simulink library "common_lib"  (R2015a)
settings: Solver=ode45  StartTime=0.0  StopTime=10.0  RelTol=1e-3
settings Model: Creator=SktUser15  LastModifiedBy=daysys

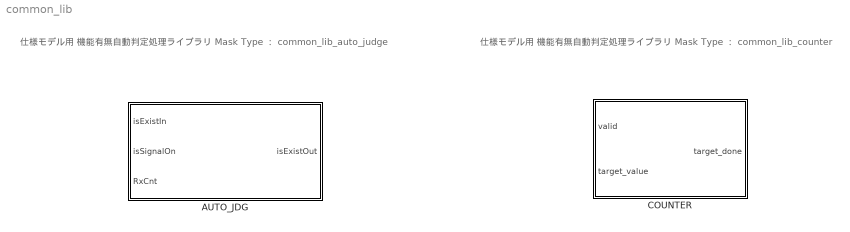
== system common_lib ==
  note: 仕様モデル用 機能有無自動判定処理ライブラリ
      | Mask Type ： common_lib_auto_judge
  note: 仕様モデル用 機能有無自動判定処理ライブラリ
      | Mask Type ： common_lib_counter
  AUTO_JDG : Subsystem  RequirementInfo={'other' '..\doc\SRS_Lib_AUTO_JDG.docx' '@Simulink_requirement_item_1' 'true' '[SRS_Lib_AUTO_JDG_Module _01-001]' '' ; 'other' '..\doc\SRS_Lib_AUTO_JDG.docx' '@Simulink_requirement_item_2' 'true' '[SRS_Lib_AUTO_JDG_Module _01-002]' '' ; 'other' '..\doc\SRS_Lib_AUTO_JDG.docx' '@Simulink_requirement_item_3' 'true' '[SRS_Lib_AUTO_JDG_Module _01-003]' '' ; 'other' '..\doc\SRS_Lib_AUTO_JDG.docx' '@Simulink_requirement_item_4' 'true' '[SRS_Lib_AUTO_JDG_Module _01-004]' '' ; 'other' '..\doc\SRS_Lib_AUTO_JDG.docx' '@Simulink_requirement_item_5' 'true' '[SRS_Lib_AUTO_JDG_Module _01-005]' '' ; 'other' '..\doc\SRS_Lib_AUTO_JDG.docx' '@Simulink_requirement_item_6' 'true' '[SRS_Lib_AUTO_JDG_Module _01-006]' '' ; 'other' '..\doc\SRS_Lib_AUTO_JDG.docx' '@Simulink_requirement_item_7' 'true' '[SRS_Lib_AUTO_JDG_Module _01-007]' '' ; 'other' '..\doc\SRS_Lib_AUTO_JDG.docx' '@Simulink_requirement_item_8' 'true' '[SRS_Lib_AUTO_JDG_Module _01-008]' '' ; 'other' '..\doc\SRS_Lib_AUTO_JDG.docx' '@Simulink_requirement_item_9' 'true' '[SRS_Lib_AUTO_JDG_Module _01-009]' '' ; 'other' '..\doc\SRS_Lib_AUTO_JDG.docx' '@Simulink_requirement_item_10' 'true' '[SRS_Lib_AUTO_JDG_Module _01-010]' '' } %GIDa_48978b64_c379_4856_88ae_7eac96266397  TreatAsAtomicUnit=on  mask(common_lib_auto_judge){JDG_TIME_CNT=[], OutMin=1, OutMax=65535, INIT_VAL=0, STEP_VAL=1}
      mask prompts: JDG_TIME_CNT "判定時間カウント値:JDG_TIME_CNT"; OutMin "Simulink:blkprm_prompts:OutputDesignMin"; OutMax "Simulink:blkprm_prompts:OutputDesignMax"; INIT_VAL "初期値"; STEP_VAL "ステップ値"
      mask help:
      | 【機能有無自動判定処理】
      | 機能有無判定信号の受信を起点として機能有無判定時間カウントを計測し、機能有無を判定します。
      | 一度、機能有りと判定した場合、それ以降機能有無判定処理を行いません。
      |
      | 入力値は、データ範囲内で使用してください。
      | 判定時間カウント値は【自動判定時間(ms)÷駆動周期(ms)】の演算結果を使用してください。
      | 判定時間カウント値はuint16型で設定してください。
      |
      | 設定値の考え方例）
      | 自動判定時間：2100ms、駆動時間：20ms
      | 判定時間カウント値 ＝ 2100ms ÷ 20ms ＝ 105
      |
      | 設定例）FUNC_JDG_TIME_CNT
      | ※機能側で”FUNC_JDG_TIME_CNT=uint16(105)”と定義済みとします。
      settings: AttributesFormatString=|
      | [isExistIn]データ範囲：True/False
      | [isSignalOn]データ範囲：True/False
      | [RxCnt]データ範囲：0～255
      | 判定時間カウント値：%<JDG_TIME_CNT>
      mask Help:
      | 【機能有無自動判定処理】
      | 機能有無判定信号の受信を起点として機能有無判定時間カウントを計測し、機能有無を判定します。
      | 一度、機能有りと判定した場合、それ以降機能有無判定処理を行いません。
      | 
      | -----------------------------------------------------------------
      | [入力]
      | inExistIn　：入力値(データ型:boolean, サイズ:[1 1], ポート番号1)
      | isSignalOn ：入力値(データ型:boolean, サイズ:[1 1], ポート番号2)
      | RxCnt      ：入力値(データ型:uint8, サイズ:[1 1], ポート番号3)
      | 
      | [出力]
      | isExistOut ：平均値(データ型:boolean, サイズ:[1 1], ポート番号1)
      | 
      | [マスクパラメータ]
      | JDG_TIME_CNT：判定時間カウント値(データ型：uint16)
      | -----------------------------------------------------------------
      mask TypeOptions OutMin: JDG_EXIST/jdgTimeCnt/OutMin
      mask TypeOptions OutMax: JDG_EXIST/jdgTimeCnt/OutMax
  COUNTER : Subsystem  TreatAsAtomicUnit=on  mask(common_lib_counter){}
      mask help:
      | 【common_lib】COUNTER v1.0
      | --------------------------------------------------------------------------------------------
      |
      | [機能概要]
      | ・カウントアップを行い、指定した回数カウントが終了するとtarget_doneはTRUEを出力します。
      | ・カウントアップ値は1です。
      | ・カウント初期値は0で固定です。
      | ・validがFALSEになると、内部のカウンタ値は0に初期化されます。
      | --------------------------------------------------------------------------------------------
      |
      | [入力]
      | 1: valid (boolean) : TRUEの間、カウント値がカウントアップします。
      | 2: target_value (uint16) : target_done検出上限値。この値までカウントアップしたらtarget_valueはTRUEを出力します。
      | [出力]
      | 1: target_done (boolean) : 初期出力FALSE。target_valueで指定した値までカウントされたとき、TRUEを出力します。
      mask Help:
      | 【common_lib】COUNTER v1.0
      | --------------------------------------------------------------------------------------------
      | 
      | [機能概要]
      | ・カウントアップを行い、指定した回数カウントが終了するとtarget_doneはTRUEを出力します。
      | ・カウントアップ値は1です。
      | ・カウント初期値は0で固定です。
      | ・validがFALSEになると、内部のカウンタ値は0に初期化されます。
      | --------------------------------------------------------------------------------------------
      | 
      | [入力]
      | 1: valid (boolean) : TRUEの間、カウント値がカウントアップします。
      | 2: target_value (uint16) : target_done検出上限値。この値までカウントアップしたらtarget_valueはTRUEを出力します。
      | [出力]
      | 1: target_done (boolean) : 初期出力FALSE。target_valueで指定した値までカウントされたとき、TRUEを出力します。

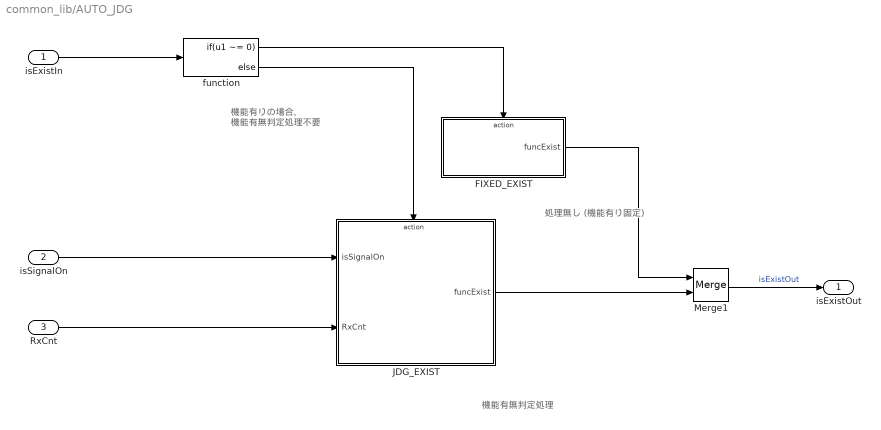
== system common_lib/AUTO_JDG ==
  note: 機能有無判定処理
  note: 処理無し
      | (機能有り固定)
  note: 機能有りの場合、
      | 機能有無判定処理不要
  isExistIn : Inport  OutDataTypeStr=boolean
      settings: AttributesFormatString=データ型：%<OutDataTypeStr>
  isSignalOn : Inport  Port=2  OutDataTypeStr=boolean
      settings: AttributesFormatString=データ型：%<OutDataTypeStr>
  RxCnt : Inport  Port=3  OutDataTypeStr=uint8
      settings: AttributesFormatString=データ型：%<OutDataTypeStr>
  FIXED_EXIST : Subsystem  TreatAsAtomicUnit=on
  JDG_EXIST : Subsystem  TreatAsAtomicUnit=on
  Merge1 : Merge  InitialOutput=false
      settings: AttributesFormatString=初期値：%<InitialOutput>
  function : If  IfExpression=u1 ~= 0
  isExistOut : Outport  OutDataTypeStr=boolean
      settings: AttributesFormatString=データ型：%<OutDataTypeStr>
  wires:
  JDG_EXIST/1(funcExist) -> Merge1/2
  function/2 -> JDG_EXIST/Action
  FIXED_EXIST/1(funcExist) -> Merge1/1
  function/1 -> FIXED_EXIST/Action
  Merge1/1 -> isExistOut/1  "isExistOut"
  isExistIn/1 -> function/1
  isSignalOn/1 -> JDG_EXIST/1(isSignalOn)
  RxCnt/1 -> JDG_EXIST/2(RxCnt)

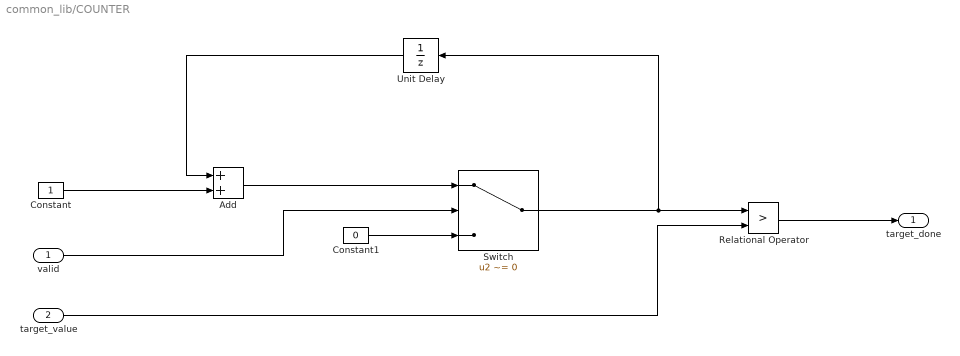
== system common_lib/COUNTER ==
  valid : Inport  OutDataTypeStr=boolean
  target_value : Inport  Port=2  OutDataTypeStr=uint16
  Add : Sum  OutDataTypeStr=uint16  RndMeth=Round  SaturateOnIntegerOverflow=on
      settings: AttributesFormatString=|
      | 整数オーバーフローで飽和 : %<SaturateOnIntegerOverflow>
      | 丸め方法 : %<RndMeth>
  Constant : Constant  OutDataTypeStr=uint16
      settings: AttributesFormatString=|
      | ----------------------------
      | 1サンプルにつき1カウントアップ
      | 出力データ型 : %<OutDataTypeStr>
  Constant1 : Constant  Value=0  OutDataTypeStr=uint16
      settings: AttributesFormatString=|
      | ----------------------------
      | valid == FALSE時に0にリセット
      | 出力データ型 : %<OutDataTypeStr>
  Relational Operator : RelationalOperator  Operator=>  OutDataTypeStr=boolean
  Switch : Switch  Criteria=u2 ~= 0  OutDataTypeStr=uint16  RndMeth=Round  SaturateOnIntegerOverflow=on
      settings: AttributesFormatString=%<RndMeth>
  Unit Delay : UnitDelay  SampleTime=-1
      settings: AttributesFormatString=初期値 : %<InitialCondition>
  target_done : Outport  OutDataTypeStr=boolean
  wires:
  valid/1 -> Switch/2
  Relational Operator/1 -> target_done/1
  Switch/1 -> Relational Operator/1, Unit Delay/1
  Constant/1 -> Add/2
  Constant1/1 -> Switch/3
  Add/1 -> Switch/1
  target_value/1 -> Relational Operator/2
  Unit Delay/1 -> Add/1

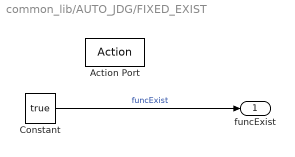
== system common_lib/AUTO_JDG/FIXED_EXIST ==
  Action Port : ActionPort  InitializeStates=reset  ActionType=then
      settings: AttributesFormatString=再開時の状態：%<InitializeStates>
  Constant : Constant  Description=TRUE：機能有り  Value=true
      settings: AttributesFormatString=%<Description>
  funcExist : Outport  InitialOutput=false
      settings: AttributesFormatString=|
      | 初期値: %<InitialOutput>
      | ディセーブル時の出力: %<OutputWhenDisabled>
  wires:
  Constant/1 -> funcExist/1  "funcExist"

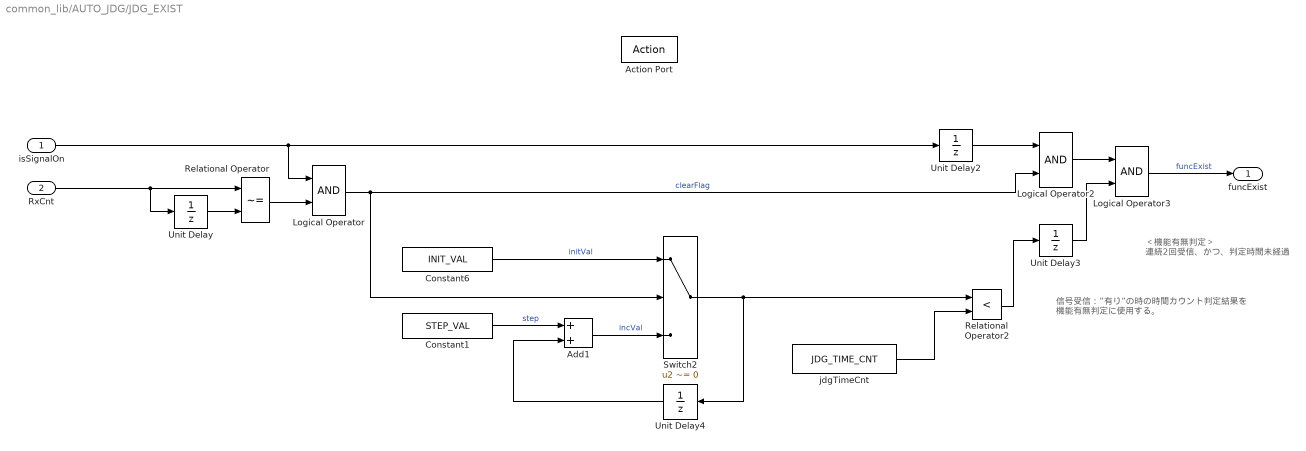
== system common_lib/AUTO_JDG/JDG_EXIST ==
  note: ＜機能有無判定＞
      | 連続2回受信、かつ、判定時間未経過
  note: 信号受信：”有り”の時の時間カウント判定結果を
      | 機能有無判定に使用する。
  isSignalOn : Inport
  RxCnt : Inport  Port=2
  Action Port : ActionPort  InitializeStates=reset  ActionType=else
      settings: AttributesFormatString=再開時の状態：%<InitializeStates>
  Add1 : Sum  SaturateOnIntegerOverflow=on  InputSameDT=on  OutDataTypeStr=Inherit: Same as first input
      settings: AttributesFormatString=|
      | 整数オーバーフローで飽和 : %<SaturateOnIntegerOverflow>
      | 入力が同じ型：%<InputSameDT>
  Constant1 : Constant  Value=STEP_VAL  OutDataTypeStr=uint16
      settings: AttributesFormatString=出力型：%<OutDataTypeStr>
  Constant6 : Constant  Value=INIT_VAL  OutDataTypeStr=uint16
      settings: AttributesFormatString=|
      | clearFlag == true時にリセット
      | 出力型：%<OutDataTypeStr>
  Logical Operator : Logic  OutDataTypeStr=boolean
  Logical Operator2 : Logic  OutDataTypeStr=boolean
  Logical Operator3 : Logic  OutDataTypeStr=boolean
  Relational Operator : RelationalOperator  Operator=~=  OutDataTypeStr=boolean  InputSameDT=on
  Relational Operator2 : RelationalOperator  Operator=<  OutDataTypeStr=boolean  InputSameDT=on
  Switch2 : Switch  Criteria=u2 ~= 0  OutDataTypeStr=uint16  InputSameDT=on
      settings: AttributesFormatString=入力が同じ型：%<InputSameDT>
  Unit Delay : UnitDelay  SampleTime=-1
      settings: AttributesFormatString=初期値：%<InitialCondition>
  Unit Delay2 : UnitDelay  InitialCondition=false  SampleTime=-1
      settings: AttributesFormatString=初期値：%<InitialCondition>
  Unit Delay3 : UnitDelay  InitialCondition=false  SampleTime=-1
      settings: AttributesFormatString=初期値：%<InitialCondition>
  Unit Delay4 : UnitDelay  InitialCondition=JDG_TIME_CNT  SampleTime=-1
      settings: AttributesFormatString=初期値 : %<InitialCondition>
  jdgTimeCnt : Constant  Value=JDG_TIME_CNT  OutMin=OutMin  OutMax=OutMax  OutDataTypeStr=uint16
      settings: AttributesFormatString=出力型：%<OutDataTypeStr>
  funcExist : Outport  InitialOutput=false
      settings: AttributesFormatString=|
      | 初期値：%<InitialOutput>
      | ディセーブル時の出力：%<OutputWhenDisabled>
  wires:
  Switch2/1 -> Unit Delay4/1, Relational Operator2/1
  Constant6/1 -> Switch2/1  "initVal"
  Add1/1 -> Switch2/3  "incVal"
  Unit Delay4/1 -> Add1/2
  Relational Operator2/1 -> Unit Delay3/1
  Constant1/1 -> Add1/1  "step"
  isSignalOn/1 -> Logical Operator/1, Unit Delay2/1
  Unit Delay2/1 -> Logical Operator2/1
  RxCnt/1 -> Relational Operator/1, Unit Delay/1
  Logical Operator/1 -> Logical Operator2/2, Switch2/2  "clearFlag"
  Logical Operator3/1 -> funcExist/1  "funcExist"
  Logical Operator2/1 -> Logical Operator3/1
  Unit Delay3/1 -> Logical Operator3/2
  Unit Delay/1 -> Relational Operator/2
  Relational Operator/1 -> Logical Operator/2
  jdgTimeCnt/1 -> Relational Operator2/2
